simulink model "prosthesis_plant"  (R2022b)
settings: Solver=ode4  StartTime=0.0  StopTime=5  FixedStep=5e-4  RelTol=1e-3
InitFcn:
  | plant = prost;
model workspace: external: MAT-File D:\repos\hand_modeling_toolbox\examples\hand_one\hand_one_model.mat (data not in the file)
values from neighbouring files (symbols this model uses):
  mdh_matrix = mdh_struct_to_matrix(mdh_default_struct, 1)    [create_model.m]    (also in create_model.mat = [0 1.57079632679 0 0 0 0 0 0 0 0 0 0.363 ... (32 elements, 8; create_model_pr_mkII_V1.m; create_model_pr_mkII_V1_7dof.m)
  prost = Finger('Index', 'type','R_RRRRRRR', 'l_links',robot_dimension)    [create_model.m]    (also in create_model_pr_mkII_V1_7dof.m)
  q_init = zeros(7,1)    [create_model.m]    (also in create_model_pr_mkII_V1_7dof.m)
  qD_init = zeros(7,1)    [create_model.m]    (also in create_model_pr_mkII_V1_7dof.m)
settings Model: Creator=ge26jow  LastModifiedBy=ge26jow
settings DebuggingCC: UnconnectedInputMsg=warning  UnconnectedOutputMsg=warning  UnconnectedLineMsg=warning
settings ModelReferenceCC: EnableRefExpFcnMdlSchedulingChecks=on
settings RTWCC: DLArmComputeVersion=19.05

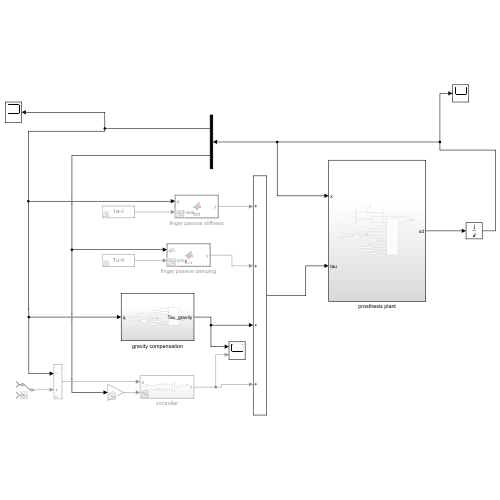
[thumbnail: Simulink's stored preview of the top-level diagram]
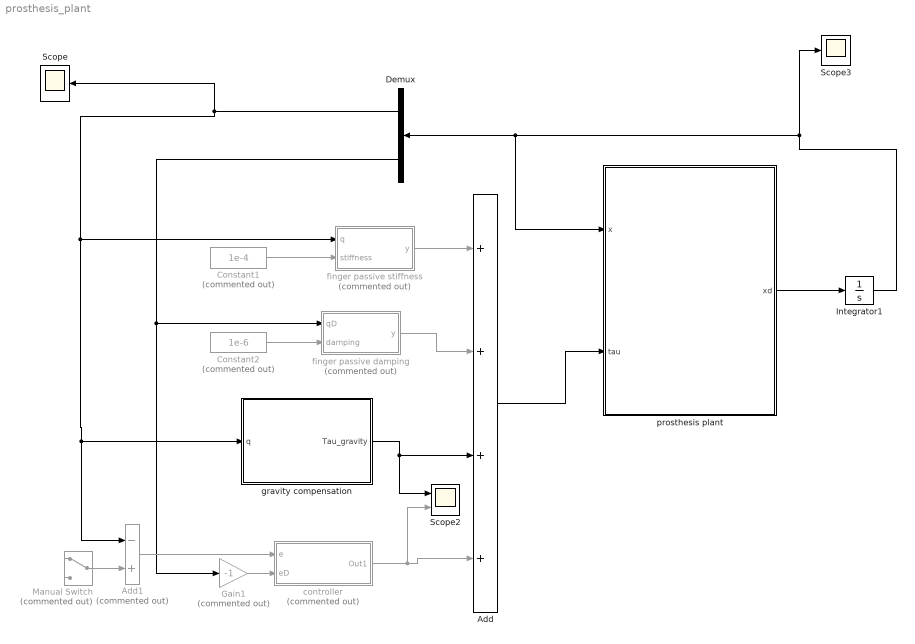
== system prosthesis_plant ==
  Add : Sum  Inputs=++++
  Add1 : Sum  Commented=on  Inputs=-+
  Constant1 : Constant  Commented=on  Value=1e-4
  Constant2 : Constant  Commented=on  Value=1e-6
  Demux : Demux  Outputs=[7,7]
  Gain1 : Gain  Commented=on  Gain=-1
  Integrator1 : Integrator  InitialCondition=[q_init;qD_init]  WrappedStateUpperValue=[pi,pi,pi,pi,1e4,1e4,1e4,1e4]  WrappedStateLowerValue=-[pi,pi,pi,pi,1e4,1e4,1e4,1e4]
  Manual Switch : ManualSwitch  Commented=on
  Scope : Scope
  Scope2 : Scope  NumInputPorts=2
  Scope3 : Scope
  controller : Subsystem  Commented=on
  finger passive damping : MATLAB Function  Commented=on  TreatAsAtomicUnit=on
  finger passive stiffness : MATLAB Function  Commented=on  TreatAsAtomicUnit=on
  gravity compensation : Subsystem
  prosthesis plant : Subsystem
  wires:
  Demux/1 -> finger passive stiffness/1(q), Add1/1, gravity compensation/1(q), Scope/1
  Add/1 -> prosthesis plant/2(tau)
  finger passive stiffness/1(y) -> Add/1
  finger passive damping/1(y) -> Add/2
  Demux/2 -> Gain1/1, finger passive damping/1(qD)
  Constant1/1 -> finger passive stiffness/2(stiffness)
  Constant2/1 -> finger passive damping/2(damping)
  gravity compensation/1(Tau_gravity) -> Add/3, Scope2/1
  Add1/1 -> controller/1(e)
  controller/1(Out1) -> Scope2/2, Add/4
  Gain1/1 -> controller/2(eD)
  Manual Switch/1 -> Add1/2
  prosthesis plant/1(xd) -> Integrator1/1
  Integrator1/1 -> Demux/1, prosthesis plant/1(x), Scope3/1

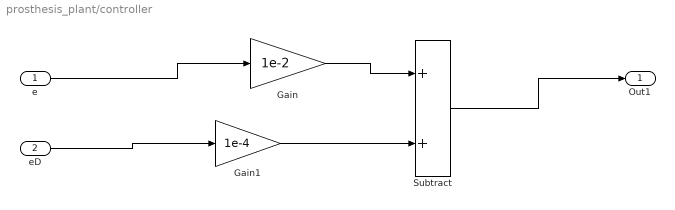
== system prosthesis_plant/controller ==
  e : Inport
  eD : Inport  Port=2
  Gain : Gain  Gain=1e-2
  Gain1 : Gain  Gain=1e-4
  Subtract : Sum
  Out1 : Outport
  wires:
  e/1 -> Gain/1
  Gain/1 -> Subtract/1
  eD/1 -> Gain1/1
  Gain1/1 -> Subtract/2
  Subtract/1 -> Out1/1

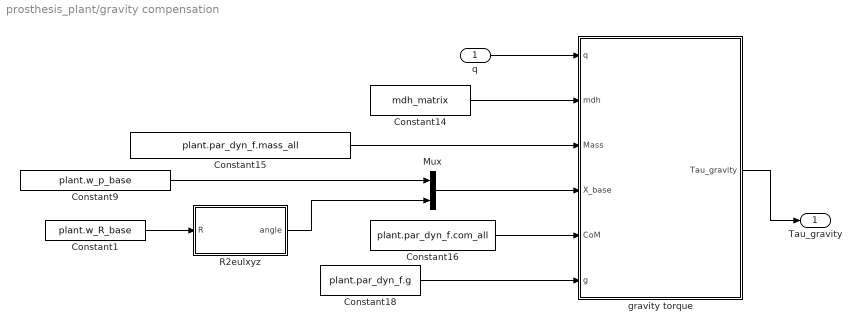
== system prosthesis_plant/gravity compensation ==
  q : Inport
  Constant1 : Constant  Value=plant.w_R_base
  Constant14 : Constant  Value=mdh_matrix
  Constant15 : Constant  Value=plant.par_dyn_f.mass_all
  Constant16 : Constant  Value=plant.par_dyn_f.com_all
  Constant18 : Constant  Value=plant.par_dyn_f.g
  Constant9 : Constant  Value=plant.w_p_base
  Mux : Mux  Inputs=[3,3]
  R2eulxyz : MATLAB Function  TreatAsAtomicUnit=on
  "gravity torque " : MATLAB Function  TreatAsAtomicUnit=on
  Tau_gravity : Outport
  wires:
  Constant14/1 -> "gravity torque "/2(mdh)
  Constant16/1 -> "gravity torque "/5(CoM)
  Mux/1 -> "gravity torque "/4(X_base)
  Constant18/1 -> "gravity torque "/6(g)
  Constant15/1 -> "gravity torque "/3(Mass)
  "gravity torque "/1(Tau_gravity) -> Tau_gravity/1
  q/1 -> "gravity torque "/1(q)
  Constant1/1 -> R2eulxyz/1(R)
  Constant9/1 -> Mux/1
  R2eulxyz/1(angle) -> Mux/2

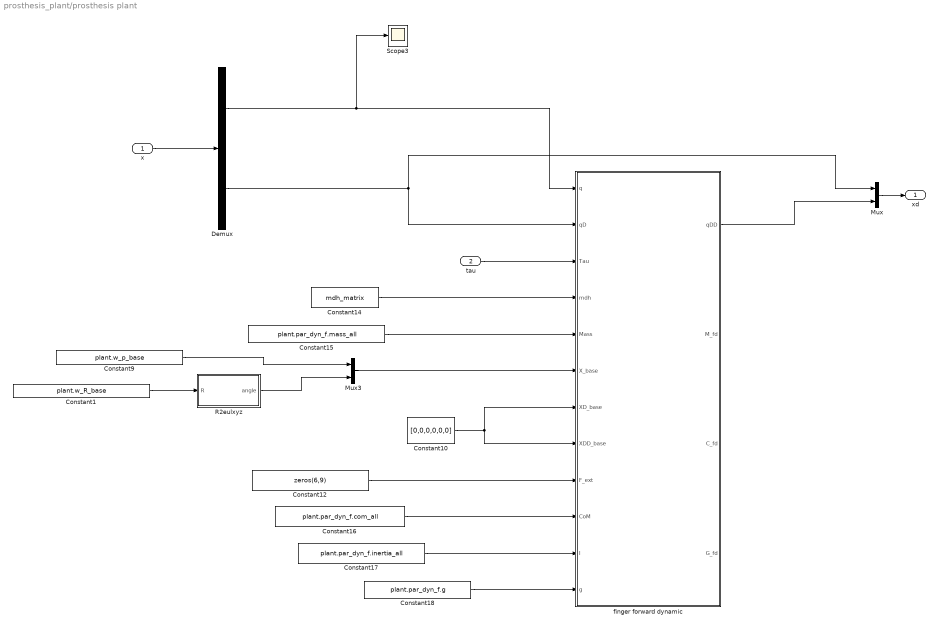
== system prosthesis_plant/prosthesis plant ==
  x : Inport
  tau : Inport  Port=2
  Constant1 : Constant  Value=plant.w_R_base
  Constant10 : Constant  Value=[0,0,0,0,0,0]
  Constant12 : Constant  Value=zeros(6,9)
  Constant14 : Constant  Value=mdh_matrix
  Constant15 : Constant  Value=plant.par_dyn_f.mass_all
  Constant16 : Constant  Value=plant.par_dyn_f.com_all
  Constant17 : Constant  Value=plant.par_dyn_f.inertia_all
  Constant18 : Constant  Value=plant.par_dyn_f.g
  Constant9 : Constant  Value=plant.w_p_base
  Demux : Demux  Outputs=[7,7]
  Mux : Mux  Inputs=2
  Mux3 : Mux  Inputs=[3,3]
  R2eulxyz : MATLAB Function  TreatAsAtomicUnit=on
  Scope3 : Scope
  finger forward dynamic : MATLAB Function  TreatAsAtomicUnit=on
  xd : Outport
  wires:
  Constant18/1 -> finger forward dynamic/12(g)
  tau/1 -> finger forward dynamic/3(Tau)
  Constant17/1 -> finger forward dynamic/11(I)
  finger forward dynamic/1(qDD) -> Mux/2
  Constant10/1 -> finger forward dynamic/7(XD_base), finger forward dynamic/8(XDD_base)
  Demux/2 -> Mux/1, finger forward dynamic/2(qD)
  Mux3/1 -> finger forward dynamic/6(X_base)
  Constant14/1 -> finger forward dynamic/4(mdh)
  Demux/1 -> Scope3/1, finger forward dynamic/1(q)
  Constant12/1 -> finger forward dynamic/9(F_ext)
  Constant15/1 -> finger forward dynamic/5(Mass)
  Constant16/1 -> finger forward dynamic/10(CoM)
  Mux/1 -> xd/1
  Constant1/1 -> R2eulxyz/1(R)
  R2eulxyz/1(angle) -> Mux3/2
  Constant9/1 -> Mux3/1
  x/1 -> Demux/1

== matlab function prosthesis_plant/prosthesis plant/finger forward dynamic ==
  data: q input; qDD output; qD input; Tau input; mdh input; Mass input; X_base input; XD_base input; XDD_base input; F_ext input; CoM input; I input; g input; M_fd output; C_fd output; G_fd output
% recursive Newton-Euler method to compute inverse dynamic with mdh
% parameters
% Input:
%     q,qD:             [n_qx1] joint states
%     Tau               [n_q] joint torque
%     mdh:              [n_q+1x4] in sequence of [alpha,a,theta,d] To be
%                       noted that the theta should exclude from mdh parameters 
%     Mass:             [n_q+1] mass vector. the first mass is the base 
%     X_base:           [6x1] eulerxyz
%     XD_base:          [6x1] translational and angular velocity
%     F_ext:            [6x1] force/moment that exerted by the environment to the endeffector frame. 
%     CoM:              [3xn_q+1] in local frame; last column is endeffector
%     I:                [6xn_q+1] in local frame with respect to center of mass. in sequence of [xx yy zz yz xz xy]
%     g:                [3x1] gravity term
% 
% Output:
%     qDD:              [n_qx1] joint acceleration 
%     M_fd:             [n_qxn_q] Mass matrix 
%     C_fd:             [n_q] velocity-dependent torque 
%     G_fd:             [n_q] gravity torque  

function [qDD,M_fd,C_fd,G_fd] = fordyn_ne_mdh(q,qD,Tau,mdh, Mass, X_base, XD_base,XDD_base, F_ext, CoM, I, g)
coder.extrinsic('invdyn_ne_mdh_mex');

n_q = length(q);
% assert(n_q == length(qD)&&n_q == length(Tau),'fordyn_ne_mdh: dimension error!');

mex = 1;


M_fd = zeros(n_q,n_q);
G_fd = zeros(n_q,1);
C_fd = zeros(n_q,1);

% gravity term
if mex
    G_fd = invdyn_ne_mdh_mex(q,zeros(n_q,1),zeros(n_q,1),mdh, Mass,...
        X_base, XD_base, XDD_base, zeros(6,1), CoM, I, g);
else
    G_fd = invdyn_ne_mdh(q,zeros(n_q,1),zeros(n_q,1),mdh, Mass,...
        X_base, XD_base, XDD_base, zeros(6,1), CoM, I, g);
end
% C term
if mex
    C_fd = invdyn_ne_mdh_mex(q,qD,zeros(n_q,1),mdh, Mass,...
        X_base, XD_base, XDD_base, zeros(6,1), CoM, I, g);
else
    C_fd = invdyn_ne_mdh(q,qD,zeros(n_q,1),mdh, Mass,...
             X_base, XD_base, XDD_base, zeros(6,1), CoM, I, g);
end
C_fd = C_fd - G_fd;

% M term
M_fd = zeros(n_q,n_q);

for i = 1:n_q
    qDD_M = zeros(n_q,1);
    qDD_M(i) = 1;
    if mex
        M_fd(:,i) = invdyn_ne_mdh_mex(q,zeros(n_q,1),qDD_M,mdh, Mass,...
            X_base, XD_base, XDD_base, zeros(6,1), CoM, I, g);
    else
        M_fd(:,i) = invdyn_ne_mdh(q,zeros(n_q,1),qDD_M,mdh, Mass,...
            X_base, XD_base, XDD_base, zeros(6,1), CoM, I, g);
    end
    M_fd(:,i) = M_fd(:,i) - G_fd;
end

% use Jacobian_geom_mdh.m to calculate geometric Jacobian
w_R_b = euler2R_XYZ(X_base(4:6));
b_J = Jacobian_geom_mdh(mdh,q);
J_ne = blkdiag(w_R_b,w_R_b)*b_J;
tau_ext = zeros(n_q,1);
for i = 1:n_q+1
    mdh_i = mdh(1:i,:);
    q_i = q(1:min(i,n_q));
    b_J_i = zeros(6,n_q);
    b_J_i(:,1:min(i,n_q)) =  Jacobian_geom_mdh(mdh_i,q_i);
    J_ne_i= blkdiag(w_R_b,w_R_b)*b_J_i;
    tau_i = J_ne_i'*F_ext(:,i+1);
    tau_ext = tau_ext + tau_i;
end


qDD = (M_fd)\(Tau + tau_ext - G_fd - C_fd);


end

== matlab function prosthesis_plant/finger passive stiffness ==
  data: q input; y output; stiffness input
function y = fcn(q,stiffness)

y = -stiffness.*q;

== matlab function prosthesis_plant/finger passive damping ==
  data: qD input; y output; damping input
function y = fcn(qD,damping)

y = -damping.*qD;

== matlab function prosthesis_plant/gravity compensation/gravity torque  ==
  data: q input; Tau_gravity output; mdh input; Mass input; X_base input; CoM input; g input
function Tau_gravity = fcn(q,mdh, Mass, X_base, CoM, g)

Tau_gravity = invdyn_ne_mdh_all_fext_gravity(q,mdh, Mass, X_base, CoM, g);

== matlab function prosthesis_plant/gravity compensation/R2eulxyz ==
  data: R input; angle output
function angle = fcn(R)

angle = R2euler_XYZ(R);

== matlab function prosthesis_plant/prosthesis plant/R2eulxyz ==
  data: R input; angle output
function angle = fcn(R)

angle = R2euler_XYZ(R);
